simulink model "Sim_Robot_mobile"  (Simulink 8.3)
settings: Solver=ode3  StartTime=0.0  StopTime=150  FixedStep=0.05  RelTol=1e-2
libraries: simulink x1
settings Model: Creator=Eric  LastModifiedBy=andes1
settings OptimizationCC: ExpressionDepthLimit=2147483647
settings DebuggingCC: FcnCallInpInsideContextMsg=EnableAllAsWarning

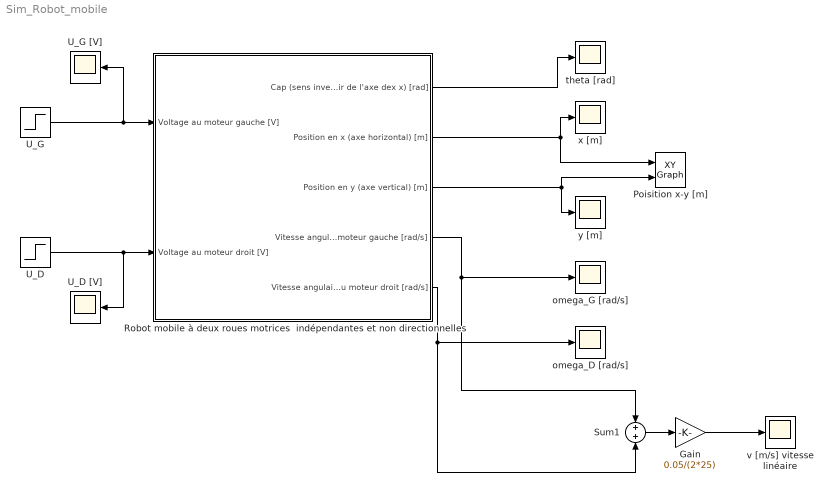
== system Sim_Robot_mobile ==
  Gain : Gain  Gain=0.05/(2*25)
  Poisition x-y [m] : simulink/Sinks/XY Graph  xmin=-4  xmax=4  ymin=-4  ymax=4  st=-1
  Robot mobile à deux roues motrices  indépendantes et non directionnelles : Subsystem
      mask Display: image('RobotImage.JPG',[5 90 85 92]);
  Sum1 : Sum
  U_D : Step  Time=0.1  After=12.5  SampleTime=0
  "U_D [V] " : Scope
      settings: TimeRange=150  YMin=0  YMax=14  SaveName=ScopeData6
  U_G : Step  Time=10  After=12  SampleTime=0
  "U_G [V] " : Scope
      settings: TimeRange=150  YMin=0  YMax=12  SaveName=ScopeData5
  omega_D [rad/s] : Scope
      settings: TimeRange=150  YMin=-20  YMax=100  SaveName=ScopeData4
  omega_G [rad/s] : Scope
      settings: TimeRange=150  YMin=-20  YMax=100  SaveName=ScopeData3
  theta [rad] : Scope
      settings: TimeRange=150  YMax=30
  v [m/s] vitesse linéaire : Scope
      settings: TimeRange=150  YMin=-0.05  YMax=0.2  SaveName=ScopeData7
  x [m] : Scope
      settings: TimeRange=150  YMin=-3  YMax=3
  y [m] : Scope
      settings: TimeRange=150  YMin=-4  YMax=1  SaveName=ScopeData2
  wires:
  Robot mobile à deux roues motrices  indépendantes et non directionnelles/2(Position en x (axe horizontal) [m]) -> Poisition x-y [m]/1, x [m]/1
  Robot mobile à deux roues motrices  indépendantes et non directionnelles/3(Position en y (axe vertical) [m]) -> Poisition x-y [m]/2, y [m]/1
  Robot mobile à deux roues motrices  indépendantes et non directionnelles/1(Cap (sens inverse horloge à partir de l'axe dex x) [rad]) -> theta [rad]/1
  Robot mobile à deux roues motrices  indépendantes et non directionnelles/4(Vitesse angulaire du moteur gauche [rad/s]) -> Sum1/1, omega_G [rad/s]/1
  Robot mobile à deux roues motrices  indépendantes et non directionnelles/5(Vitesse angulaire du moteur droit [rad/s]) -> Sum1/2, omega_D [rad/s]/1
  U_G/1 -> Robot mobile à deux roues motrices  indépendantes et non directionnelles/1(Voltage au moteur gauche [V]), "U_G [V] "/1
  Gain/1 -> v [m/s] vitesse linéaire/1
  Sum1/1 -> Gain/1
  U_D/1 -> "U_D [V] "/1, Robot mobile à deux roues motrices  indépendantes et non directionnelles/2(Voltage au moteur droit [V])

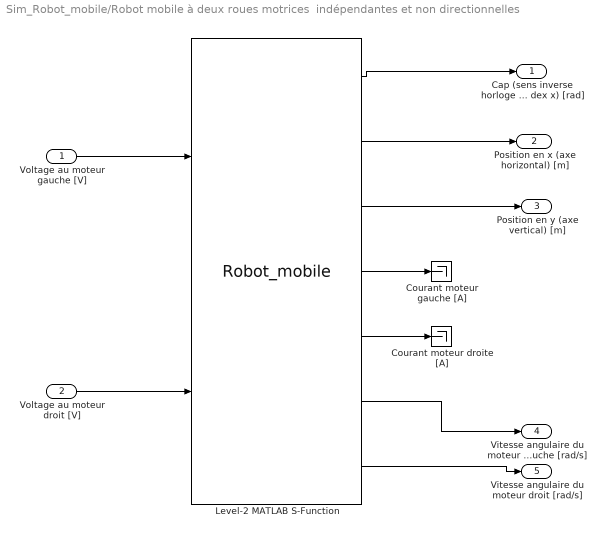
== system Sim_Robot_mobile/Robot mobile à deux roues motrices  indépendantes et non directionnelles ==
  Voltage au moteur gauche [V] : Inport
  Voltage au moteur droit [V] : Inport  Port=2
  Courant moteur droite [A] : Terminator
  Courant moteur gauche [A] : Terminator
  Level-2 MATLAB S-Function : M-S-Function  FunctionName=Robot_mobile
  Cap (sens inverse horloge à partir de l'axe dex x) [rad] : Outport
  Position en x (axe horizontal) [m] : Outport  Port=2
  Position en y (axe vertical) [m] : Outport  Port=3
  Vitesse angulaire du moteur gauche [rad/s] : Outport  Port=4
  Vitesse angulaire du moteur droit [rad/s] : Outport  Port=5
  wires:
  Voltage au moteur droit [V]/1 -> Level-2 MATLAB S-Function/2
  Voltage au moteur gauche [V]/1 -> Level-2 MATLAB S-Function/1
  Level-2 MATLAB S-Function/1 -> Cap (sens inverse horloge à partir de l'axe dex x) [rad]/1
  Level-2 MATLAB S-Function/2 -> Position en x (axe horizontal) [m]/1
  Level-2 MATLAB S-Function/3 -> Position en y (axe vertical) [m]/1
  Level-2 MATLAB S-Function/6 -> Vitesse angulaire du moteur gauche [rad/s]/1
  Level-2 MATLAB S-Function/7 -> Vitesse angulaire du moteur droit [rad/s]/1
  Level-2 MATLAB S-Function/4 -> Courant moteur gauche [A]/1
  Level-2 MATLAB S-Function/5 -> Courant moteur droite [A]/1
